simulink library "data_driven_lib_sys"  (R2024a)
settings: Solver=VariableStepAuto  StartTime=0.0  StopTime=10.0  RelTol=1e-3
undefined symbols (not defined in the file or in its folder): ActiveScenario, otter_params
libraries: mssSimulink x1
settings Model: Creator=luka  LastModifiedBy=luka

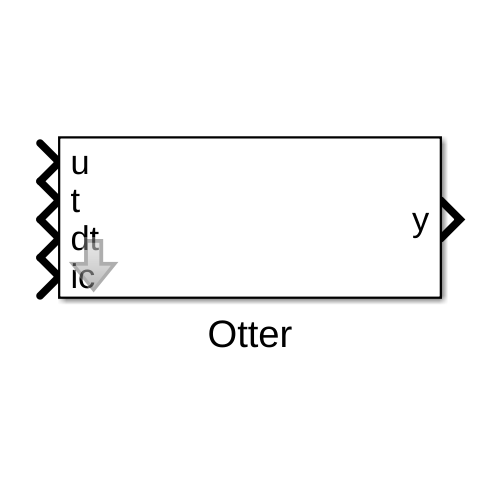
[thumbnail: Simulink's stored preview of the top-level diagram]
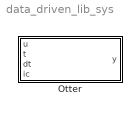
== system data_driven_lib_sys ==
  Otter : Subsystem  Tag=__cs_slx_sys  mask{params=otter_params, merged_params=ActiveScenario.Params}
      mask prompts: params "Environment parameters"

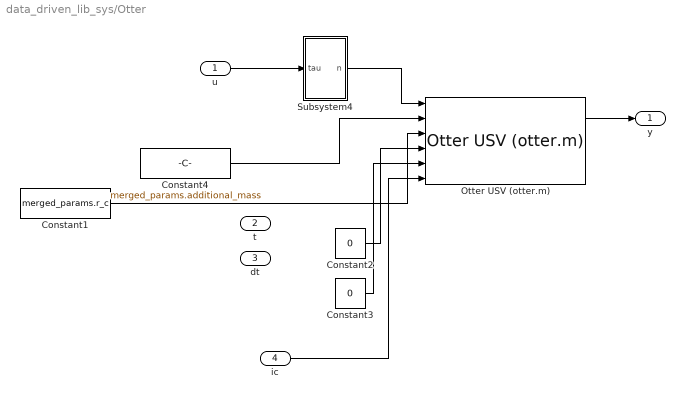
== system data_driven_lib_sys/Otter ==
  u : Inport  PortDimensions=2
  t : Inport  Port=2
  dt : Inport  Port=3
  ic : Inport  Port=4
  Constant1 : Constant  Value=merged_params.r_c
  Constant2 : Constant  Value=0
  Constant3 : Constant  Value=0
  Constant4 : Constant  Value=merged_params.additional_mass
  Otter USV (otter.m) : mssSimulink/Marine craft models/Otter USV (otter.m)  SystemSampleTime=-1  VariantActivationTime=update diagram  AllowFlexibleInterface=on  Latency=0  AutoFrameSizeCalculation=off
  Subsystem4 : Subsystem
  y : Outport  PortDimensions=12
  wires:
  ic/1 -> Otter USV (otter.m)/6
  Constant3/1 -> Otter USV (otter.m)/5
  Constant2/1 -> Otter USV (otter.m)/4
  Constant1/1 -> Otter USV (otter.m)/3
  Constant4/1 -> Otter USV (otter.m)/2
  Subsystem4/1(n) -> Otter USV (otter.m)/1
  u/1 -> Subsystem4/1(tau)
  Otter USV (otter.m)/1 -> y/1

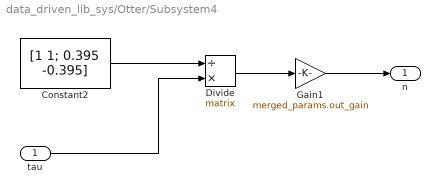
== system data_driven_lib_sys/Otter/Subsystem4 ==
  tau : Inport
  Constant2 : Constant  Value=[1 1; 0.395 -0.395]
  Divide : Product  Inputs=/*  Multiplication=Matrix(*)
  Gain1 : Gain  Gain=merged_params.out_gain
  n : Outport
  wires:
  Gain1/1 -> n/1
  tau/1 -> Divide/2
  Divide/1 -> Gain1/1
  Constant2/1 -> Divide/1
